simulink model "harness_Antony_Lab_4"  (R2023b)
settings: Solver=ode45  StartTime=0.0  StopTime=100  FixedStep=1/10  RelTol=1e-3
InitFcn:
  | init_fn()
values from neighbouring files (symbols this model uses):
  MAX_TORQUE_REVERSE = 40    [init_fn.m]
undefined symbols (not defined in the file or in its folder): sigbuilder_block
libraries: simulink x11, arduinolib x10
settings Model: NumberOfSteps=20  PacingRate=10  Creator=Jacopo Sini  LastModifiedBy=Utilisateur
settings OptimizationCC: ReuseModelBlockBuffer=off
settings DebuggingCC: UnconnectedInputMsg=warning  UnconnectedOutputMsg=warning  UnconnectedLineMsg=warning
settings ModelReferenceCC: EnableRefExpFcnMdlSchedulingChecks=on
settings RTWCC: DLArmComputeVersion=19.05

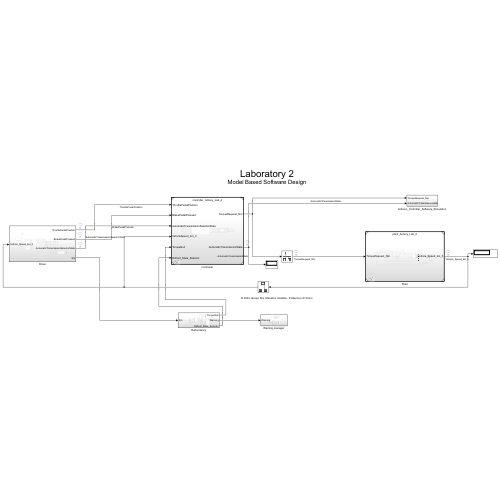
[thumbnail: Simulink's stored preview of the top-level diagram]
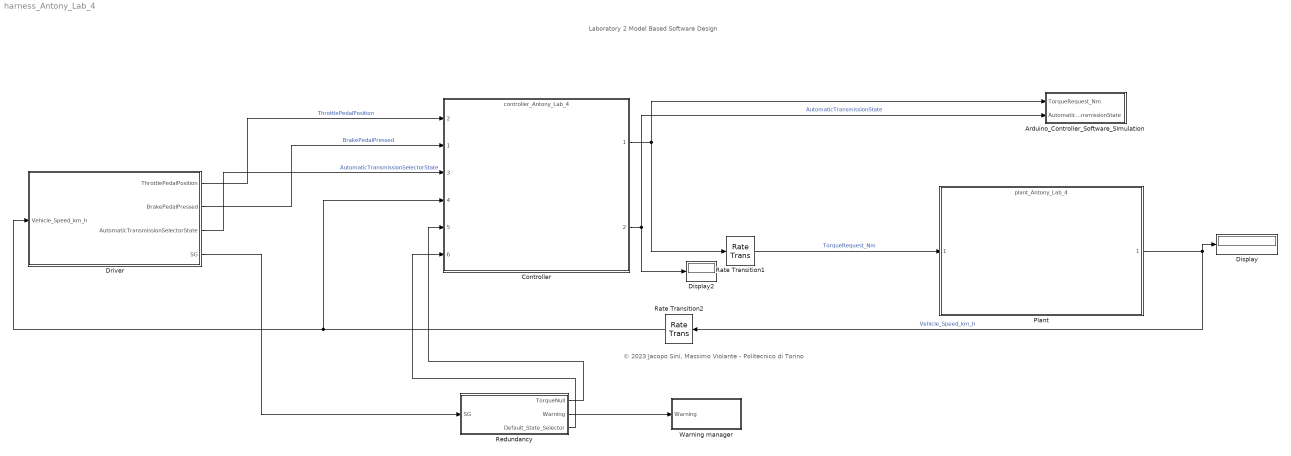
== system harness_Antony_Lab_4 ==
  note: © 2023 Jacopo Sini, Massimo Violante - Politecnico di Torino
  note: Laboratory 2
      | Model Based Software Design
  Arduino_Controller_Software_SImulation : Subsystem
  Controller : ModelReference  ModelNameDialog=controller_Antony_Lab_4  SimulationMode=Normal  ModelReferenceVersion=5.74
      settings: PortSchema="{\"entries\":[{\"content\":{\"sides\":[{\"content\":{\"connectorIds\":[\"In2\",\"In1\",\"In3\",\"In4\",\"In5\",\"In6\"]},\"type\":\"ConnectorPlacement.EquallySpacedRectSide\",\"uuid\":\"5e260b81-e1ce-497c-8572-ac5c2182ee27\"},{\"content\":{\"connectorIds\":[\"Out1\",\"Out2\"],\"side\":\"RIGHT\"},\"type\":\"ConnectorPlacement.EquallySpacedRectSide\",\"uuid\":\"4325f63c-e453-4c79-ab01-1476da99aa25\"},{\"content\":{\"side\":\"TOP\"},\"type\":\"ConnectorPlacement.EquallySpacedRectSide\",\"uuid\":\"dba88bac-0f95-4a98-ba3b-c40df5616f56\"}]},\"type\":\"ConnectorPlacement.EquallySpacedConnector\",\"uuid\":\"6943e10d-f3b0-4fd8-a142-b6b49e651f90\"}],\"packageUris\":[\"http://schema.mathworks.com/mf0/Connector/R2020b\"],\"version\":\"1.0\"}"
  Display : Display
  Display2 : Display
  Driver : Subsystem
  Plant : ModelReference  ModelNameDialog=plant_Antony_Lab_4  SimulationMode=Normal  ModelReferenceVersion=3.19
  Rate Transition1 : RateTransition
  Rate Transition2 : RateTransition
  Redundancy : Subsystem
  Warning manager : Subsystem
  wires:
  Plant/1 -> Display/1, Rate Transition2/1  "Vehicle_Speed_km_h"
  Rate Transition2/1 -> Driver/1(Vehicle_Speed_km_h), Controller/4
  Controller/2 -> Arduino_Controller_Software_SImulation/2(AutomaticTransmissionState), Display2/1  "AutomaticTransmissionState"
  Driver/1(ThrottlePedalPosition) -> Controller/2  "ThrottlePedalPosition"
  Driver/2(BrakePedalPressed) -> Controller/1  "BrakePedalPressed"
  Driver/3(AutomaticTransmissionSelectorState) -> Controller/3  "AutomaticTransmissionSelectorState"
  Driver/4(SG) -> Redundancy/1(SG)
  Redundancy/1(TorqueNull) -> Controller/5
  Redundancy/2(Warning) -> Warning manager/1(Warning)
  Rate Transition1/1 -> Plant/1  "TorqueRequest_Nm"
  Redundancy/3(Default_State_Selector) -> Controller/6
  Controller/1 -> Arduino_Controller_Software_SImulation/1(TorqueRequest_Nm), Rate Transition1/1

== system harness_Antony_Lab_4/Arduino_Controller_Software_SImulation ==
  TorqueRequest_Nm : Inport
  AutomaticTransmissionState : Inport  Port=2
  Torque_Light_Block : Subsystem
  Transmission_Light_Block : Subsystem
  wires:
  TorqueRequest_Nm/1 -> Torque_Light_Block/1(TorqueRequest_Nm)
  AutomaticTransmissionState/1 -> Transmission_Light_Block/1(AutomaticTransmissionState)

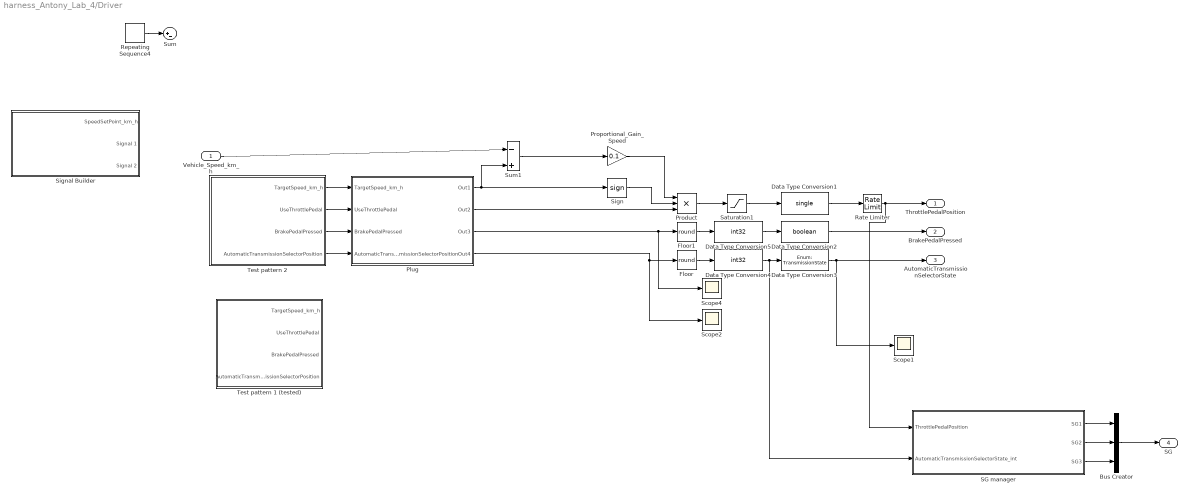
== system harness_Antony_Lab_4/Driver ==
  Vehicle_Speed_km_h : Inport
  Bus Creator : BusCreator  Inputs=3
  Data Type Conversion1 : DataTypeConversion  OutDataTypeStr=single  SaturateOnIntegerOverflow=off  RndMeth=Floor  LockScale=on
  Data Type Conversion2 : DataTypeConversion  OutDataTypeStr=boolean  SaturateOnIntegerOverflow=off  RndMeth=Floor  LockScale=on
  Data Type Conversion3 : DataTypeConversion  OutDataTypeStr=Enum: TransmissionState  SaturateOnIntegerOverflow=off  RndMeth=Floor  LockScale=on
  Data Type Conversion4 : DataTypeConversion  OutDataTypeStr=int32  SaturateOnIntegerOverflow=off  RndMeth=Floor  LockScale=on
  Data Type Conversion5 : DataTypeConversion  OutDataTypeStr=int32  SaturateOnIntegerOverflow=off  RndMeth=Floor  LockScale=on
  Floor : Rounding  Operator=round
  Floor1 : Rounding  Operator=round
  Plug : Subsystem
  Product : Product  Inputs=3
  Proportional_Gain_Speed : Gain  Gain=0.1
  Rate Limiter : RateLimiter  RisingSlewLimit=0.5  SampleTimeMode=inherited
  Repeating Sequence4 : simulink/Sources/Repeating Sequence  rep_seq_t=[0 10 500]  rep_seq_y=[10 0 0]
  SG manager : Subsystem
  Saturation1 : Saturate  UpperLimit=1  LowerLimit=0
  Scope1 : Scope
  Scope2 : Scope
  Scope4 : Scope
  Sign : Signum
  Signal Builder : Subsystem  Tag=STV Subsys  LoadFcn=sigbuilder_block('load');  StartFcn=sigbuilder_block('start');  StopFcn=sigbuilder_block('stop');  ClipboardFcn=sigbuilder_block('clipboard');  mask(Sigbuilder block){tuvar=[0:10]}
      mask help: Simulink:masks:SigbuilderBlock_MD
      mask init:
      | if ~strcmp(get_param(bdroot(gcbh),'SimulationStatus'),'stopped') tuvar = sigbuilder_block('maskInit'); end
      settings: CopyFcn=sigbuilder_block('copy');  DeleteFcn=sigbuilder_block('delete');  ModelCloseFcn=sigbuilder_block('modelClose');  PreSaveFcn=sigbuilder_block('preSave');  PauseFcn=sigbuilder_block('pause');  ContinueFcn=sigbuilder_block('continue');  NameChangeFcn=sigbuilder_block('namechange');  OpenFcn=sigbuilder_block('open',[0 84 2240 1072 ]);  CloseFcn=sigbuilder_block('close');
      mask Display: plot(0, 0, 100, 100,[2, 2, 32, 32, 2], [68, 8, 8, 68, 68],[32, 2], [38, 38], [32, 19, 2],[53, 60, 44], [32, 17, 17, 2],[16, 16, 31, 31]);txt = getActiveGroup(gcbh);text(2, 100, txt,'verticalAlignment', 'top');
  Sum : Sum  Inputs=|+-
  Sum1 : Sum  Inputs=|-+
  Test pattern 1 (tested) : Subsystem
  Test pattern 2 : Subsystem
  ThrottlePedalPosition : Outport
  BrakePedalPressed : Outport  Port=2
  AutomaticTransmissionSelectorState : Outport  Port=3  OutDataTypeStr=Enum: TransmissionState
  SG : Outport  Port=4
  wires:
  Data Type Conversion1/1 -> Rate Limiter/1
  Data Type Conversion2/1 -> BrakePedalPressed/1
  Data Type Conversion3/1 -> AutomaticTransmissionSelectorState/1, Scope1/1
  Floor/1 -> Data Type Conversion4/1
  Data Type Conversion4/1 -> SG manager/2(AutomaticTransmissionSelectorState_int), Data Type Conversion3/1
  Floor1/1 -> Data Type Conversion5/1
  Data Type Conversion5/1 -> Data Type Conversion2/1
  Product/1 -> Saturation1/1
  Sum1/1 -> Proportional_Gain_Speed/1
  Sign/1 -> Product/2
  Saturation1/1 -> Data Type Conversion1/1
  Rate Limiter/1 -> SG manager/1(ThrottlePedalPosition), ThrottlePedalPosition/1
  Repeating Sequence4/1 -> Sum/1
  Vehicle_Speed_km_h/1 -> Sum1/1
  Proportional_Gain_Speed/1 -> Product/1
  Plug/1(Out1) -> Sum1/2, Sign/1
  Plug/3(Out3) -> Scope4/1, Floor1/1
  Plug/4(Out4) -> Scope2/1, Floor/1
  Plug/2(Out2) -> Product/3
  Test pattern 2/1(TargetSpeed_km_h) -> Plug/1(TargetSpeed_km_h)
  Test pattern 2/2(UseThrottlePedal) -> Plug/2(UseThrottlePedal)
  Test pattern 2/3(BrakePedalPressed) -> Plug/3(BrakePedalPressed)
  Test pattern 2/4(AutomaticTransmissionSelectorPosition) -> Plug/4(AutomaticTransmissionSelectorPosition)
  SG manager/1("SG1 ") -> Bus Creator/1
  Bus Creator/1 -> SG/1
  SG manager/2(SG2) -> Bus Creator/2
  SG manager/3(SG3) -> Bus Creator/3

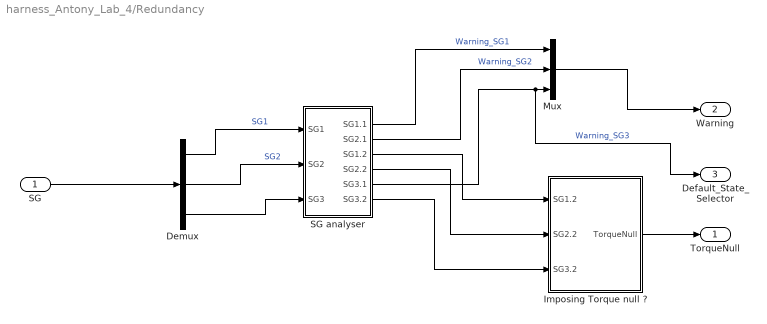
== system harness_Antony_Lab_4/Redundancy ==
  SG : Inport
  Demux : Demux  Outputs=3
  Imposing Torque null ? : Subsystem
  Mux : Mux  Inputs=3
  SG analyser : Subsystem
  TorqueNull : Outport
  Warning : Outport  Port=2
  Default_State_Selector : Outport  Port=3
  wires:
  SG/1 -> Demux/1
  Imposing Torque null ?/1(TorqueNull) -> TorqueNull/1
  Demux/1 -> SG analyser/1(SG1)  "SG1"
  Demux/2 -> SG analyser/2(SG2)  "SG2"
  SG analyser/1(SG1.1) -> Mux/1  "Warning_SG1"
  SG analyser/2(SG2.1) -> Mux/2  "Warning_SG2"
  SG analyser/3(SG1.2) -> Imposing Torque null ?/1(SG1.2)
  SG analyser/4(SG2.2) -> Imposing Torque null ?/2(SG2.2)
  Mux/1 -> Warning/1
  Demux/3 -> SG analyser/3(SG3)
  SG analyser/5(SG3.1) -> Default_State_Selector/1, Mux/3  "Warning_SG3"
  SG analyser/6(SG3.2) -> Imposing Torque null ?/3(SG3.2)

== system harness_Antony_Lab_4/Warning manager ==
  note: Warnings
      | Each warning respectively to a safety goal is a boolean .
      | - 0 : No warning emitted
      | - 1 : A warning is emitted
  Warning : Inport
  Demux : Demux  Outputs=3
  Warning display : Scope  NumInputPorts=3
  wires:
  Warning/1 -> Demux/1
  Demux/1 -> Warning display/1  "SG1"
  Demux/2 -> Warning display/2  "SG2"
  Demux/3 -> Warning display/3  "SG3"

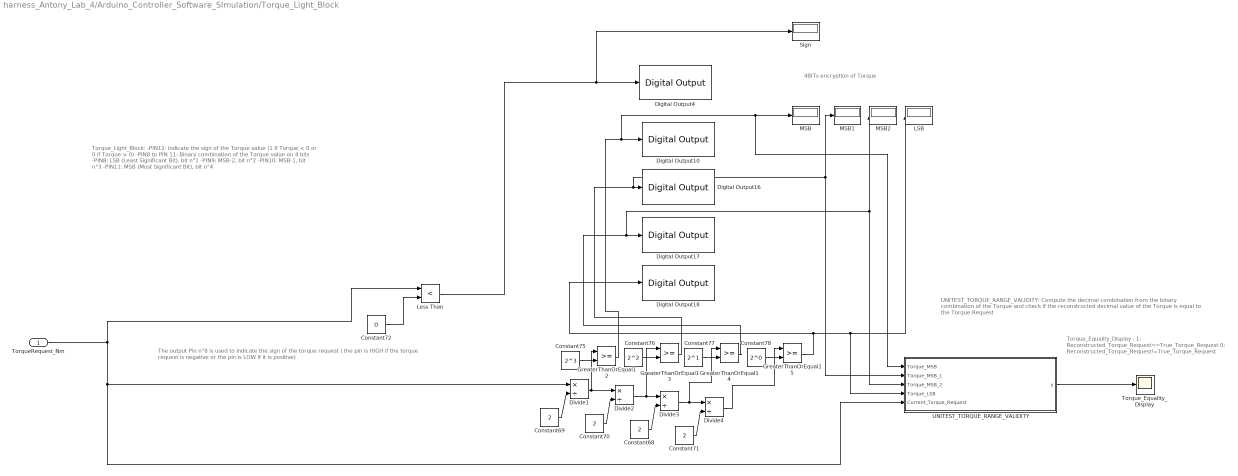
== system harness_Antony_Lab_4/Arduino_Controller_Software_SImulation/Torque_Light_Block ==
  note: The output Pin n°8 is used to indicate the sign of the torque request ( the pin is HIGH if the torque request is negative or the pin is LOW if it is positive)
  note: 4BITs encryption of Torque
  note: Torque_Light_Block:
      | -PIN12: indicate the sign of the Torque value (1 if Torque < 0 or 0 if Torque > 0)
      | -PIN8 to PIN 11: Binary combination of the Torque value on 4 bits
      | -PIN8: LSB (Least Significant Bit), bit n°1
      | -PIN9: MSB-2, bit n°2
      | -PIN10: MSB-1, bit n°3
      | -PIN11: MSB (Most Significant Bit), bit n°4
  note: UNITEST_TORQUE_RANGE_VALIDITY:
      | Compute the decimal combination from the binary combination of the Torque and check if the reconstructed decimal value of the Torque is equal to the Torque Request
  note: Torque_Equality_Display :
      | 1: Reconstructed_Torque_Request==True_Torque_Request
      | 0: Reconstructed_Torque_Request!=True_Torque_Request
  TorqueRequest_Nm : Inport
  Constant{68..71} (4 alike) : Constant  Value=2
  Constant72 : Constant  Value=0
  Constant75 : Constant  Value=2^3
  Constant76 : Constant  Value=2^2
  Constant77 : Constant  Value=2^1
  Constant78 : Constant  Value=2^0
  Digital Output10 : arduinolib/Digital Output  pinNumber=11  Direction=output  blockPlatform=arduino
  Digital Output16 : arduinolib/Digital Output  pinNumber=10  Direction=output  blockPlatform=arduino
  Digital Output17 : arduinolib/Digital Output  pinNumber=9  Direction=output  blockPlatform=arduino
  Digital Output18 : arduinolib/Digital Output  pinNumber=8  Direction=output  blockPlatform=arduino
  Digital Output4 : arduinolib/Digital Output  pinNumber=12  Direction=output  blockPlatform=arduino
  Divide{1..4} (4 alike) : Product  Inputs=*/
  GreaterThanOrEqual{12..15} (4 alike) : RelationalOperator  OutDataTypeStr=boolean  RndMeth=Simplest  InputSameDT=off
  LSB : Display
  Less Than : RelationalOperator  Operator=<  OutDataTypeStr=boolean  RndMeth=Simplest  InputSameDT=off
  MSB : Display
  MSB1 : Display
  MSB2 : Display
  Sign : Display
  Torque_Equality_Display : Scope
  UNITEST_TORQUE_RANGE_VALIDITY : MATLAB Function  TreatAsAtomicUnit=on
  wires:
  Divide4/1 -> GreaterThanOrEqual15/1
  TorqueRequest_Nm/1 -> Less Than/1, Divide1/1, UNITEST_TORQUE_RANGE_VALIDITY/5(Current_Torque_Request)
  Divide1/1 -> GreaterThanOrEqual12/1, Divide2/1
  Constant68/1 -> Divide3/2
  Constant69/1 -> Divide1/2
  Constant78/1 -> GreaterThanOrEqual15/2
  Constant77/1 -> GreaterThanOrEqual14/2
  Less Than/1 -> Sign/1, Digital Output4/1
  Constant70/1 -> Divide2/2
  Constant72/1 -> Less Than/2
  Constant76/1 -> GreaterThanOrEqual13/2
  GreaterThanOrEqual12/1 -> UNITEST_TORQUE_RANGE_VALIDITY/1(Torque_MSB), MSB/1, Digital Output10/1
  Constant71/1 -> Divide4/2
  GreaterThanOrEqual13/1 -> UNITEST_TORQUE_RANGE_VALIDITY/2(Torque_MSB_1), MSB1/1, Digital Output16/1
  GreaterThanOrEqual14/1 -> MSB2/1, UNITEST_TORQUE_RANGE_VALIDITY/3(Torque_MSB_2), Digital Output17/1
  GreaterThanOrEqual15/1 -> Digital Output18/1, UNITEST_TORQUE_RANGE_VALIDITY/4(Torque_LSB), LSB/1
  Divide3/1 -> GreaterThanOrEqual14/1, Divide4/1
  Constant75/1 -> GreaterThanOrEqual12/2
  Divide2/1 -> GreaterThanOrEqual13/1, Divide3/1
  UNITEST_TORQUE_RANGE_VALIDITY/1(y) -> Torque_Equality_Display/1

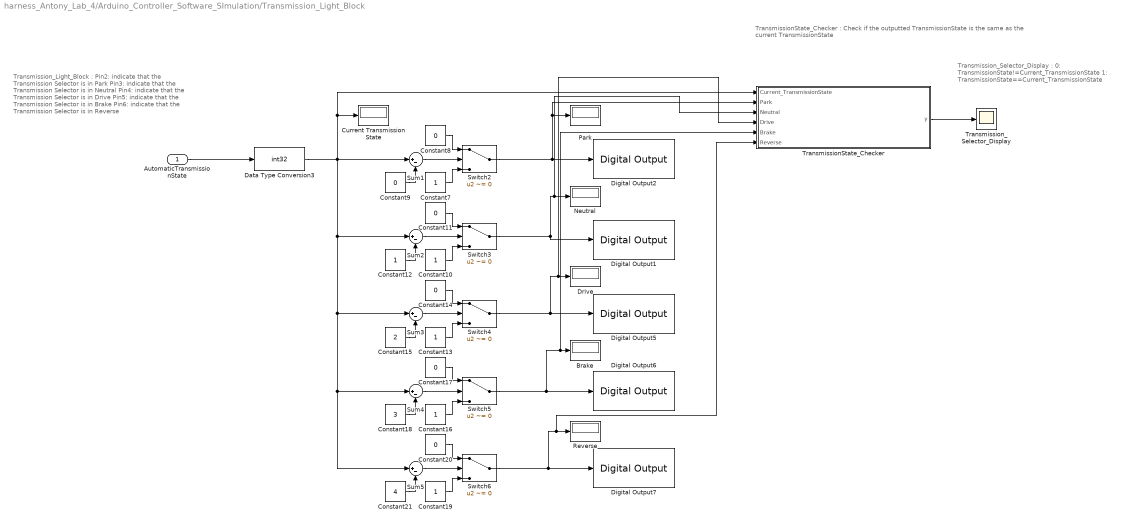
== system harness_Antony_Lab_4/Arduino_Controller_Software_SImulation/Transmission_Light_Block ==
  note: Transmission_Light_Block :
      | Pin2: indicate that the Transmission Selector is in Park
      | Pin3: indicate that the Transmission Selector is in Neutral
      | Pin4: indicate that the Transmission Selector is in Drive
      | Pin5: indicate that the Transmission Selector is in Brake
      | Pin6: indicate that the Transmission Selector is in Reverse
  note: Transmission_Selector_Display :
      | 0: TransmissionState!=Current_TransmissionState
      | 1: TransmissionState==Current_TransmissionState
  note: TransmissionState_Checker :
      | Check if the outputted TransmissionState is the same as the current TransmissionState
  AutomaticTransmissionState : Inport
  Brake : Display
  Constant{7,10,12..13,16,19} (6 alike) : Constant
  Constant{8..9,11,14,17,20} (6 alike) : Constant  Value=0
  Constant15 : Constant  Value=2
  Constant18 : Constant  Value=3
  Constant21 : Constant  Value=4
  Current Transmission State : Display
  Data Type Conversion3 : DataTypeConversion  OutDataTypeStr=int32  SaturateOnIntegerOverflow=off  RndMeth=Floor  LockScale=on
  Digital Output1 : arduinolib/Digital Output  pinNumber=3  Direction=output  blockPlatform=arduino
  Digital Output2 : arduinolib/Digital Output  pinNumber=2  Direction=output  blockPlatform=arduino
  Digital Output5 : arduinolib/Digital Output  pinNumber=4  Direction=output  blockPlatform=arduino
  Digital Output6 : arduinolib/Digital Output  pinNumber=5  Direction=output  blockPlatform=arduino
  Digital Output7 : arduinolib/Digital Output  pinNumber=6  Direction=output  blockPlatform=arduino
  Drive : Display
  Neutral : Display
  Park : Display
  Reverse : Display
  Sum{1..5} (5 alike) : Sum  Inputs=|+-
  Switch{2..6} (5 alike) : Switch  Criteria=u2 ~= 0  Threshold=MAX_TORQUE_REVERSE  SaturateOnIntegerOverflow=off  InputSameDT=off
  TransmissionState_Checker : MATLAB Function  TreatAsAtomicUnit=on
  Transmission_Selector_Display : Scope
  wires:
  Sum4/1 -> Switch5/2
  Constant7/1 -> Switch2/3
  Sum2/1 -> Switch3/2
  Constant15/1 -> Sum3/2
  Sum3/1 -> Switch4/2
  Constant8/1 -> Switch2/1
  AutomaticTransmissionState/1 -> Data Type Conversion3/1
  Constant12/1 -> Sum2/2
  Constant18/1 -> Sum4/2
  Constant10/1 -> Switch3/3
  Constant11/1 -> Switch3/1
  Constant13/1 -> Switch4/3
  Constant14/1 -> Switch4/1
  Sum5/1 -> Switch6/2
  Switch3/1 -> TransmissionState_Checker/3(Neutral), Neutral/1, Digital Output1/1
  Constant17/1 -> Switch5/1
  Switch4/1 -> TransmissionState_Checker/4(Drive), Drive/1, Digital Output5/1
  Switch2/1 -> TransmissionState_Checker/2(Park), Park/1, Digital Output2/1
  Switch5/1 -> TransmissionState_Checker/5(Brake), Brake/1, Digital Output6/1
  Constant21/1 -> Sum5/2
  Sum1/1 -> Switch2/2
  Switch6/1 -> TransmissionState_Checker/6(Reverse), Reverse/1, Digital Output7/1
  Constant20/1 -> Switch6/1
  Constant16/1 -> Switch5/3
  Constant19/1 -> Switch6/3
  Constant9/1 -> Sum1/2
  Data Type Conversion3/1 -> TransmissionState_Checker/1(Current_TransmissionState), Current Transmission State/1, Sum5/1, Sum4/1, Sum3/1, Sum2/1, Sum1/1
  TransmissionState_Checker/1(y) -> Transmission_Selector_Display/1

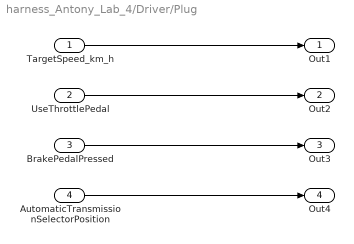
== system harness_Antony_Lab_4/Driver/Plug ==
  TargetSpeed_km_h : Inport
  UseThrottlePedal : Inport  Port=2
  BrakePedalPressed : Inport  Port=3
  AutomaticTransmissionSelectorPosition : Inport  Port=4
  Out1 : Outport
  Out2 : Outport  Port=2
  Out3 : Outport  Port=3
  Out4 : Outport  Port=4
  wires:
  TargetSpeed_km_h/1 -> Out1/1
  UseThrottlePedal/1 -> Out2/1
  BrakePedalPressed/1 -> Out3/1
  AutomaticTransmissionSelectorPosition/1 -> Out4/1

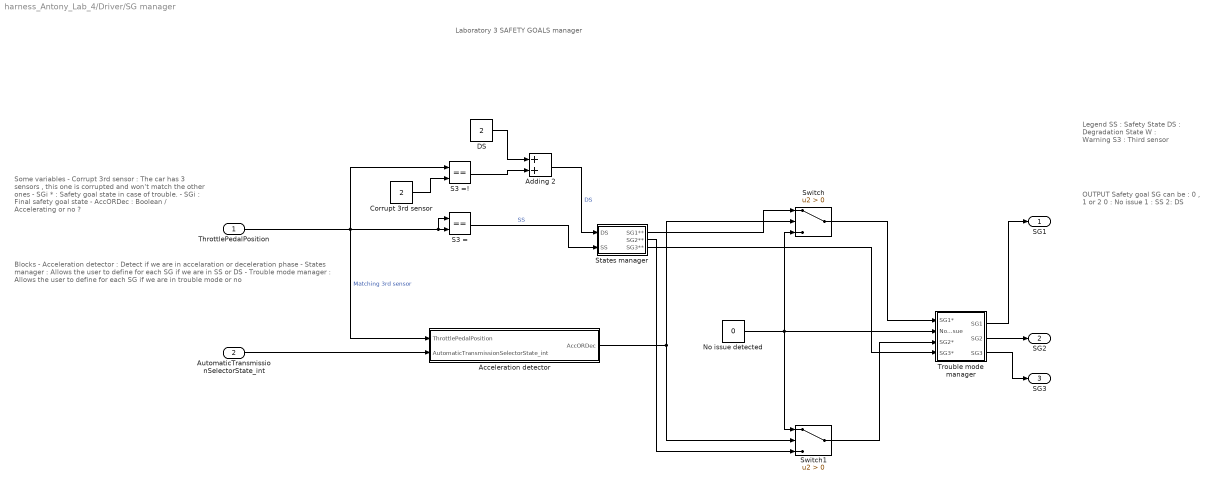
== system harness_Antony_Lab_4/Driver/SG manager ==
  note: Legend
      | SS : Safety State
      | DS : Degradation State
      | W : Warning
      | S3 : Third sensor
  note: Laboratory 3
      | SAFETY GOALS manager
  note: OUTPUT
      | Safety goal SG can be : 0 , 1 or 2
      | 0 : No issue
      | 1 : SS
      | 2: DS
  note: Some variables
      | - Corrupt 3rd sensor : The car has 3 sensors , this one is corrupted and won't match the other ones
      | - SGi * : Safety goal state in case of trouble.
      | - SGi : Final safety goal state
      | - AccORDec : Boolean / Accelerating or no ?
  note: Blocks
      | - Acceleration detector : Detect if we are in accelaration or deceleration phase
      | - States manager : Allows the user to define for each SG if we are in SS or DS
      | - Trouble mode manager : Allows the user to define for each SG if we are in trouble mode or no
  ThrottlePedalPosition : Inport
  AutomaticTransmissionSelectorState_int : Inport  Port=2
  Acceleration detector : Subsystem
  Adding 2 : Sum
  "Corrupt 3rd sensor " : Constant  Value=2
  DS : Constant  Value=2
  No issue detected : Constant  Value=0
  S3 = : RelationalOperator  Operator===  OutDataTypeStr=boolean  RndMeth=Simplest  InputSameDT=off
  "S3 =! " : RelationalOperator  Operator===  OutDataTypeStr=boolean  RndMeth=Simplest  InputSameDT=off
  States manager : Subsystem
  Switch : Switch  Criteria=u2 > Threshold  SaturateOnIntegerOverflow=off  InputSameDT=off
  Switch1 : Switch  Criteria=u2 > Threshold  SaturateOnIntegerOverflow=off  InputSameDT=off
  Trouble mode manager : Subsystem
  "SG1 " : Outport
  SG2 : Outport  Port=2
  SG3 : Outport  Port=3
  wires:
  "Corrupt 3rd sensor "/1 -> "S3 =! "/2
  No issue detected/1 -> Switch/3, Trouble mode manager/2(No_issue), Switch1/1
  ThrottlePedalPosition/1 -> Acceleration detector/1(ThrottlePedalPosition), S3 =/1, S3 =/2, "S3 =! "/1  "Matching 3rd sensor"
  "S3 =! "/1 -> Adding 2/2
  DS/1 -> Adding 2/1
  Acceleration detector/1(AccORDec) -> Switch1/2, Switch/2
  AutomaticTransmissionSelectorState_int/1 -> Acceleration detector/2(AutomaticTransmissionSelectorState_int)
  Adding 2/1 -> States manager/1(DS)  "DS"
  S3 =/1 -> States manager/2(SS)  "SS"
  States manager/1(SG1**) -> Switch/1
  States manager/2(SG2**) -> Switch1/3
  Switch/1 -> Trouble mode manager/1(SG1*)
  Switch1/1 -> Trouble mode manager/3(SG2*)
  Trouble mode manager/1(SG1) -> "SG1 "/1
  Trouble mode manager/2(SG2) -> SG2/1
  States manager/3(SG3**) -> Trouble mode manager/4(SG3*)
  Trouble mode manager/3(SG3) -> SG3/1

== system harness_Antony_Lab_4/Driver/Signal Builder ==
  Demux : Demux  Tag=STV Demux  Outputs=3
      settings: DisplayOption=none
  FromWs : FromWorkspace  Tag=STV FromWs  VariableName=tuvar
      SigBuilderData=|
      | common.afterFinalStr = 'Extrapolate'
      | common.sampleTime = 0
      | dataSet.timeRange = [0 500]
      | dataSet.name = 'Group 1'
      | sbobj.Groups.Name = 'Group 1'
      | sbobj.Groups.Signals(1).Name = 'SpeedSetPoint_km_h'
      | sbobj.Groups.Signals(1).XData = [0 2.165 2.165 6 6 500]
      | sbobj.Groups.Signals(1).YData = [0 0 1 1 0 0]
      | sbobj.Groups.Signals(2).Name = 'Signal 1'
      | sbobj.Groups.Signals(2).XData = [0 0.5 0.5 1 1 1.5 1.5 2 2 2.5 2.5 3 ... (2000 elements, 1x2000)]
      | sbobj.Groups.Signals(2).YData = [2 2 0 0 2 2 0 0 2 2 0 0 ... (2000 elements, 1x2000)]
      | sbobj.Groups.Signals(3).Name = 'Signal 2'
      | sbobj.Groups.Signals(3).XData = [0 250 250 500]
      | sbobj.Groups.Signals(3).YData = [0 0 1 1]
      | sbobj.Groups.TimeRange = [0 500]
  SpeedSetPoint_km_h : Outport  Tag=STV Outport
  Signal 1 : Outport  Tag=STV Outport  Port=2
  Signal 2 : Outport  Tag=STV Outport  Port=3
  wires:
  Demux/1 -> SpeedSetPoint_km_h/1
  FromWs/1 -> Demux/1
  Demux/2 -> Signal 1/1
  Demux/3 -> Signal 2/1

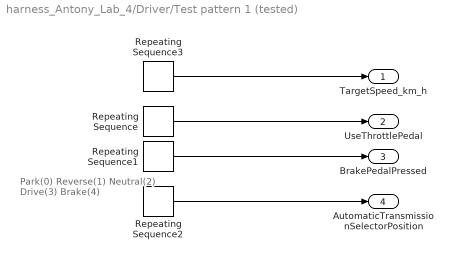
== system harness_Antony_Lab_4/Driver/Test pattern 1 (tested) ==
  note: Park(0)
      | Reverse(1)
      | Neutral(2)
      | Drive(3)
      | Brake(4)
  Repeating Sequence : simulink/Sources/Repeating Sequence  rep_seq_t=[0 3.9 4 500]  rep_seq_y=[0 0 1 1]
  Repeating Sequence1 : simulink/Sources/Repeating Sequence  rep_seq_t=[0 2.999 3 49.9 50.0 52.0 52.1 500]  rep_seq_y=[1 1 0 0 1 1 0 0]
  Repeating Sequence2 : simulink/Sources/Repeating Sequence  rep_seq_t=[0 1.999 2 10 49.9 50.0 500]  rep_seq_y=[0 0 4 4 4 1 1]
  Repeating Sequence3 : simulink/Sources/Repeating Sequence  rep_seq_t=[0 3.9 4 29.9 30 39.9 40 52.9 53 500]  rep_seq_y=[0 0 90 90 60 60 0 0 -20 -20]
  TargetSpeed_km_h : Outport
  UseThrottlePedal : Outport  Port=2
  BrakePedalPressed : Outport  Port=3
  AutomaticTransmissionSelectorPosition : Outport  Port=4
  wires:
  Repeating Sequence2/1 -> AutomaticTransmissionSelectorPosition/1
  Repeating Sequence/1 -> UseThrottlePedal/1
  Repeating Sequence1/1 -> BrakePedalPressed/1
  Repeating Sequence3/1 -> TargetSpeed_km_h/1

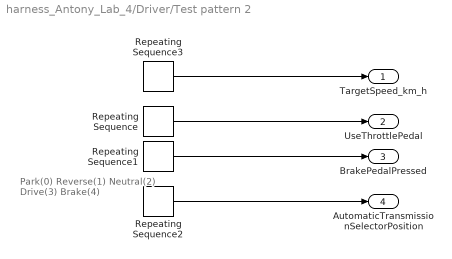
== system harness_Antony_Lab_4/Driver/Test pattern 2 ==
  note: Park(0)
      | Reverse(1)
      | Neutral(2)
      | Drive(3)
      | Brake(4)
  Repeating Sequence : simulink/Sources/Repeating Sequence  rep_seq_t=[0 3.9 4 500]  rep_seq_y=[0 0 1 1]
  Repeating Sequence1 : simulink/Sources/Repeating Sequence  rep_seq_t=[0 2.999 3 49.9 80.0 82.0 92.1 500]  rep_seq_y=[1 1 0 0 1 1 0 0]
  Repeating Sequence2 : simulink/Sources/Repeating Sequence  rep_seq_t=[0 1.999 2 10 79.9 80.0 500]  rep_seq_y=[0 2 3 4 3 2 1]
  Repeating Sequence3 : simulink/Sources/Repeating Sequence  rep_seq_t=[0 3.9 4 29.9 30 39.9 40 82.9 83 500]  rep_seq_y=[0 0 90 90 60 60 0 0 -20 -20]
  TargetSpeed_km_h : Outport
  UseThrottlePedal : Outport  Port=2
  BrakePedalPressed : Outport  Port=3
  AutomaticTransmissionSelectorPosition : Outport  Port=4
  wires:
  Repeating Sequence2/1 -> AutomaticTransmissionSelectorPosition/1
  Repeating Sequence/1 -> UseThrottlePedal/1
  Repeating Sequence1/1 -> BrakePedalPressed/1
  Repeating Sequence3/1 -> TargetSpeed_km_h/1

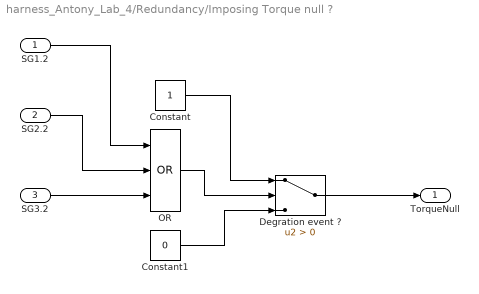
== system harness_Antony_Lab_4/Redundancy/Imposing Torque null ? ==
  SG1.2 : Inport
  SG2.2 : Inport  Port=2
  SG3.2 : Inport  Port=3
  Constant : Constant
  Constant1 : Constant  Value=0
  Degration event ? : Switch  Criteria=u2 > Threshold  SaturateOnIntegerOverflow=off  InputSameDT=off
  OR : Logic  Operator=OR  Inputs=3  IconShape=distinctive  AllPortsSameDT=off  OutDataTypeStr=boolean
  TorqueNull : Outport
  wires:
  OR/1 -> Degration event ?/2
  Constant1/1 -> Degration event ?/3
  Degration event ?/1 -> TorqueNull/1
  Constant/1 -> Degration event ?/1
  SG2.2/1 -> OR/2
  SG1.2/1 -> OR/1
  SG3.2/1 -> OR/3

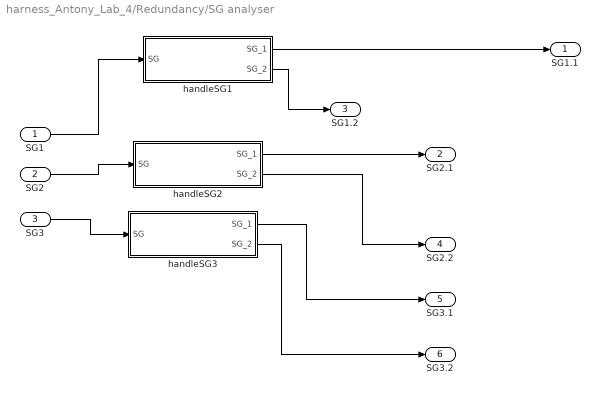
== system harness_Antony_Lab_4/Redundancy/SG analyser ==
  SG1 : Inport
  SG2 : Inport  Port=2
  SG3 : Inport  Port=3
  handleSG1 : MATLAB Function  TreatAsAtomicUnit=on
  handleSG2 : MATLAB Function  TreatAsAtomicUnit=on
  handleSG3 : MATLAB Function  TreatAsAtomicUnit=on
  SG1.1 : Outport
  SG2.1 : Outport  Port=2
  SG1.2 : Outport  Port=3
  SG2.2 : Outport  Port=4
  SG3.1 : Outport  Port=5
  SG3.2 : Outport  Port=6
  wires:
  SG2/1 -> handleSG2/1(SG)
  handleSG2/2(SG_2) -> SG2.2/1
  handleSG1/2(SG_2) -> SG1.2/1
  handleSG2/1(SG_1) -> SG2.1/1
  SG1/1 -> handleSG1/1(SG)
  handleSG1/1(SG_1) -> SG1.1/1
  SG3/1 -> handleSG3/1(SG)
  handleSG3/1(SG_1) -> SG3.1/1
  handleSG3/2(SG_2) -> SG3.2/1

== system harness_Antony_Lab_4/Driver/SG manager/Acceleration detector ==
  ThrottlePedalPosition : Inport
  AutomaticTransmissionSelectorState_int : Inport  Port=2
  1 acc | 0 dec : Switch  Criteria=u2 > Threshold  SaturateOnIntegerOverflow=off  InputSameDT=off
  Brake mode ? : RelationalOperator  Operator===  OutDataTypeStr=boolean  RndMeth=Simplest  InputSameDT=off
  Brake number : Constant  Value=4
  "acc or dec ? B mode " : simulink/Logic and Bit Operations/Compare To Constant  relop=>  const=1/3  OutDataTypeStr=boolean
  "acc or dec ? Other modes " : simulink/Logic and Bit Operations/Compare To Constant  relop=>  const=0  OutDataTypeStr=boolean
  AccORDec : Outport
  wires:
  ThrottlePedalPosition/1 -> "acc or dec ? B mode "/1, "acc or dec ? Other modes "/1
  Brake mode ?/1 -> 1 acc | 0 dec/2  "SS"
  AutomaticTransmissionSelectorState_int/1 -> Brake mode ?/2
  Brake number/1 -> Brake mode ?/1
  1 acc | 0 dec/1 -> AccORDec/1  "In trouble mode : SG1 and SG2 are opposit"
  "acc or dec ? Other modes "/1 -> 1 acc | 0 dec/3
  "acc or dec ? B mode "/1 -> 1 acc | 0 dec/1

== system harness_Antony_Lab_4/Driver/SG manager/States manager ==
  DS : Inport
  SS : Inport  Port=2
  "SG1 : DS or SS" : ManualSwitch
  "SG2 : DS or SS" : ManualSwitch
  "SG3 : DS or SS" : ManualSwitch  CurrentSetting=0
  SG1** : Outport
  SG2** : Outport  Port=2
  SG3** : Outport  Port=3
  wires:
  "SG2 : DS or SS"/1 -> SG2**/1
  "SG1 : DS or SS"/1 -> SG1**/1
  "SG3 : DS or SS"/1 -> SG3**/1
  SS/1 -> "SG3 : DS or SS"/2, "SG1 : DS or SS"/2, "SG2 : DS or SS"/2
  DS/1 -> "SG3 : DS or SS"/1, "SG2 : DS or SS"/1, "SG1 : DS or SS"/1

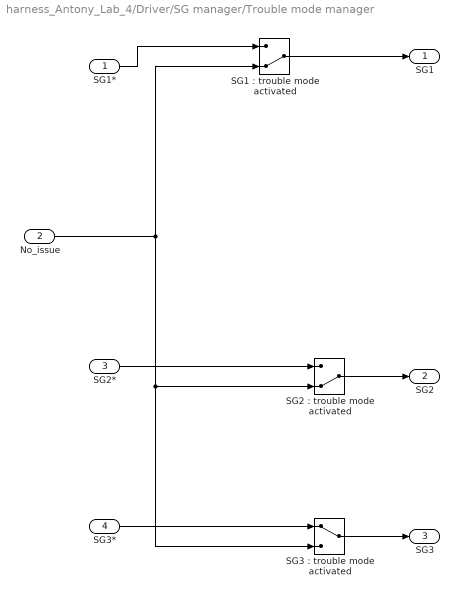
== system harness_Antony_Lab_4/Driver/SG manager/Trouble mode manager ==
  SG1* : Inport
  No_issue : Inport  Port=2
  SG2* : Inport  Port=3
  SG3* : Inport  Port=4
  "SG1 : trouble mode activated" : ManualSwitch  CurrentSetting=0
  "SG2 : trouble mode activated" : ManualSwitch  CurrentSetting=0
  "SG3 : trouble mode activated" : ManualSwitch
  SG1 : Outport
  SG2 : Outport  Port=2
  SG3 : Outport  Port=3
  wires:
  SG2*/1 -> "SG2 : trouble mode activated"/1
  SG1*/1 -> "SG1 : trouble mode activated"/1
  "SG2 : trouble mode activated"/1 -> SG2/1
  "SG1 : trouble mode activated"/1 -> SG1/1
  No_issue/1 -> "SG3 : trouble mode activated"/2, "SG2 : trouble mode activated"/2, "SG1 : trouble mode activated"/2
  SG3*/1 -> "SG3 : trouble mode activated"/1
  "SG3 : trouble mode activated"/1 -> SG3/1

== matlab function harness_Antony_Lab_4/Redundancy/SG analyser/handleSG2 ==
  data: SG input; SG_1 output; SG_2 output
function [SG_1, SG_2] = handleSG(SG)
    % Initialize the outputs
    SG_1 = 0;
    SG_2 = 0;

    % Check the value of SG and set outputs accordingly
    if isempty(SG)
        % SG is null, return SG_1 = 0 and SG_2 = 0
        SG_1 = 0;
        SG_2 = 0;
    elseif SG == 1
        % SG is 1, return SG_1 = 1 and SG_2 = 0
        SG_1 = 1;
        SG_2 = 0;
    elseif SG == 2
        % SG is 2, return SG_1 = 0 and SG_2 = 2
        SG_1 = 0;
        SG_2 = 2;
    else
        % SG is neither 1 nor 2, return SG_1 = 0 and SG_2 = 0
        SG_1 = 0;
        SG_2 = 0;
    end
end

== matlab function harness_Antony_Lab_4/Redundancy/SG analyser/handleSG1 ==
  data: SG input; SG_1 output; SG_2 output
function [SG_1, SG_2] = handleSG(SG)
    % Initialize the outputs
    SG_1 = 0;
    SG_2 = 0;

    % Check the value of SG and set outputs accordingly
    if isempty(SG)
        % SG is null, return SG_1 = 0 and SG_2 = 0
        SG_1 = 0;
        SG_2 = 0;
    elseif SG == 1
        % SG is 1, return SG_1 = 1 and SG_2 = 0
        SG_1 = 1;
        SG_2 = 0;
    elseif SG == 2
        % SG is 2, return SG_1 = 0 and SG_2 = 2
        SG_1 = 0;
        SG_2 = 2;
    else
        % SG is neither 1 nor 2, return SG_1 = 0 and SG_2 = 0
        SG_1 = 0;
        SG_2 = 0;
    end
end

== matlab function harness_Antony_Lab_4/Redundancy/SG analyser/handleSG3 ==
  data: SG input; SG_1 output; SG_2 output
function [SG_1, SG_2] = handleSG(SG)
    % Initialize the outputs
    SG_1 = 0;
    SG_2 = 0;

    % Check the value of SG and set outputs accordingly
    if isempty(SG)
        % SG is null, return SG_1 = 0 and SG_2 = 0
        SG_1 = 0;
        SG_2 = 0;
    elseif SG == 1
        % SG is 1, return SG_1 = 1 and SG_2 = 0
        SG_1 = 1;
        SG_2 = 0;
    elseif SG == 2
        % SG is 2, return SG_1 = 0 and SG_2 = 2
        SG_1 = 0;
        SG_2 = 2;
    else
        % SG is neither 1 nor 2, return SG_1 = 0 and SG_2 = 0
        SG_1 = 0;
        SG_2 = 0;
    end
end

== matlab function harness_Antony_Lab_4/Arduino_Controller_Software_SImulation/Torque_Light_Block/UNITEST_TORQUE_RANGE_VALIDITY ==
  data: Torque_MSB input; Torque_MSB_1 input; Torque_MSB_2 input; Torque_LSB input; Current_Torque_Request input; y output
function y = fcn(Torque_MSB, Torque_MSB_1, Torque_MSB_2, Torque_LSB, Current_Torque_Request)
    %% Binary/Decimal conversion of the Reconstructed Torque Request value
    Reconstructed_Torque_Request = Torque_MSB*8 + Torque_MSB_1*4 + Torque_MSB_2*2 + Torque_LSB;
    %% Computation of the real Reconstructed_Torque_Request
    Reconstructed_Torque_Request = Reconstructed_Torque_Request + (Current_Torque_Request-Reconstructed_Torque_Request);
    %% If the reconstructed Torque Request value is equal to the true Torque Request then u = "true", otherwise u = "false"
    if Reconstructed_Torque_Request==Current_Torque_Request
        u = 1;
    else
        u = 0;
    end
    %% Output the value of u
y = u;

== matlab function harness_Antony_Lab_4/Arduino_Controller_Software_SImulation/Transmission_Light_Block/TransmissionState_Checker ==
  data: Current_TransmissionState input; Park input; Neutral input; Drive input; Brake input; Reverse input; y output
function y = fcn(Current_TransmissionState, Park, Neutral, Drive, Brake, Reverse)
%% TransmissionState Test
u = 0;
if Park==1
    TransmissionState = 0;
elseif Neutral==1
    TransmissionState = 1;
elseif Drive==1
    TransmissionState = 2;
elseif Brake==1
    TransmissionState = 3;
else
    TransmissionState = 4; %%Reverse
end
%% Current_TransmissionState and TransmissionState equality test
if TransmissionState==Current_TransmissionState
    u = 1;
end
%% Output "1" if TransmissionState==Current_TransmissionState else "0"
y = u;
